simulink model "m3dscope"  (Simulink 8.4)
settings: Solver=ode45  StartTime=0.0  StopTime=10.0  RelTol=1e-3
settings Model: Creator=gcampa  LastModifiedBy=gcampa  CovHtmlReporting=off  CovSFcnEnable=on
settings DataIOCC: SaveFormat=StructureWithTime  SignalLoggingSaveFormat=Dataset  SaveOutput=off  SignalLogging=off  DSMLogging=off  SaveTime=off
settings OptimizationCC: ExpressionDepthLimit=128
settings DebuggingCC: UnderspecifiedInitializationDetection=Simplified  MergeDetectMultiDrivingBlocksExec=error  SolverPrmCheckMsg=none  FcnCallInpInsideContextMsg=EnableAllAsError  FrameProcessingCompatibilityMsg=error  StateNameClashWarn=none
settings HardwareCC: ProdBitPerPointer=64  ProdLargestAtomicFloat=Float  ProdIntDivRoundTo=Zero  ProdEndianess=LittleEndian  ProdHWDeviceType=Specified
settings GRTTargetCC: CombineOutputUpdateFcns=on  GRTInterface=off
settings hdlcc: HDLCActiveTab=48

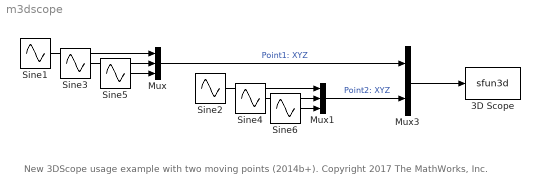
== system m3dscope ==
  note: New 3DScope usage example with two moving points (2014b+). Copyright 2017 The MathWorks, Inc.
  3D Scope : M-S-Function  LoadFcn=if exist('sfun3d','file'), sfun3d([],'LoadBlock'); end  FunctionName=sfun3d  Parameters=ax,T,np,cp,gd,ls,mk,mx,hd,tb  mask(3D Graph){np=2, ax=[-3 3 -3 3 -3 3], mx=1e4, T=0.1, cp=[3 2 1], gd=on, hd=off, tb=off, ls=-, mk=none}
      mask prompts: np "Number of moving points (lines)"; ax "Range: [xmin xmax  ymin ymax zmin zmax]"; mx "Max number of points in each line"; T "Sampling Time"; cp "Camera position (use [0 0 1] for 2D XY view)"; gd "Grid (on|off)"; hd "HeadMarkers (on|off)"; tb "Toolbar (on|off)"; ls "LineStyle"; mk "LineMarker"
      mask help:
      | This block plots the position of several points in the XYZ space. The input contains the coordinates of all the points (x1,y1,z1,x2,y2,z2,...).
      | The number of moving points (lines), the XYZ ranges, sampling time, camera position, and grid (among other things) can be set as mask parameters.
      settings: CopyFcn=if exist('sfun3d','file'), sfun3d([],'CopyBlock'); end  DeleteFcn=if exist('sfun3d','file'), sfun3d([],'DeleteBlock'); end  NameChangeFcn=if exist('sfun3d','file'), sfun3d([],'NameChange'); end
      mask Help:
      | This block plots the position of several points in the XYZ space. The input contains the coordinates of all the points (x1,y1,z1,x2,y2,z2,...).
      | The number of moving points (lines), the XYZ ranges, sampling time, camera position, and grid (among other things) can be set as mask parameters.
      mask TypeOptions ls: - | -- | : | -. | none
      mask TypeOptions mk: none | . | + | o | * | x | square | diamond | v | ^ | > | < | pentagram | hexagram
      mask Display: t=linspace(0,2*pi,50); plot(sin(2*t),sin(3*t+pi/2));
  Mux : Mux  Inputs=3
  Mux1 : Mux  Inputs=3
  Mux3 : Mux  Inputs=2
  Sine1 : Sin  SampleTime=0
  Sine2 : Sin  Amplitude=2  Frequency=2  SampleTime=0
  Sine3 : Sin  Phase=pi/2  SampleTime=0
  Sine4 : Sin  Amplitude=2  Frequency=2  Phase=pi/2  SampleTime=0
  Sine5 : Sin  Amplitude=1.5  Frequency=1.2  Phase=pi/2  SampleTime=0
  Sine6 : Sin  Amplitude=2.5  Frequency=2.2  Phase=pi/2  SampleTime=0
  wires:
  Mux/1 -> Mux3/1  "Point1: XYZ"
  Sine1/1 -> Mux/1
  Sine3/1 -> Mux/2
  Sine5/1 -> Mux/3
  Mux1/1 -> Mux3/2  "Point2: XYZ"
  Sine2/1 -> Mux1/1
  Sine6/1 -> Mux1/3
  Sine4/1 -> Mux1/2
  Mux3/1 -> 3D Scope/1
